simulink model "WEankle_controllerMaarten_2018"  (R2018b)
settings: Solver=FixedStepDiscrete  StartTime=0.0  StopTime=inf  FixedStep=sampleTime  RelTol=1e-3
PreLoadFcn:
  | init
undefined symbols (not defined in the file or in its folder): DiscIntNeverNeededParam, forceplate, Joint_params, sampleTime
libraries: simulink x21, WE2_library x9, dspsigops x6, dspfdesign x3
(part 1 of 4)
settings Model: TCT_ExtModeMexArgs=[130 89 233 2 1 1],16842768  SimulationMode=external  Creator=symbitron  LastModifiedBy=u0088756
settings DataIOCC: LimitDataPoints=on  SaveFormat=StructureWithTime
settings OptimizationCC: LocalBlockOutputs=off
settings DebuggingCC: AllowSymbolicDim=off  SFUnexpectedBacktrackingDiag=warning  SFNoUnconditionalDefaultTransitionDiag=warning  SFExecutionAtInitializationDiag=none
settings HardwareCC: ProdBitPerSizeT=32  ProdBitPerPtrDiffT=32  ProdWordSize=32  ProdHWDeviceType=Specified
settings ModelReferenceCC: PropagateSignalLabelsOutOfModel=off
settings SFSimCC: SimUseLocalCustomCode=off
settings RTWCC: Description=TwinCAT Target  SystemTargetFile=TwinCAT.tlc  GenCodeOnly=on  MakeCommand=make_tct  TemplateMakefile=tct_msbuild.tmf  GenerateReport=on  RTWUseLocalCustomCode=off  TargetLang=C++
settings CodeAppCC: StateflowObjectComments=on
settings STFCustomTargetCC: CompOptLevelCompliant=on  MATLABClassNameForMDSCustomization=Simulink.SoftwareTarget.TargetSpecificTriggerConfigurationBase  GRTInterface=on  SystemTargetFile=TwinCAT.tlc
settings ConfigComp: CovMetricSettings=dw  CovSaveCumulativeToWorkspaceVar=on  CovSaveSingleToWorkspaceVar=on  CovExternalEMLEnable=off

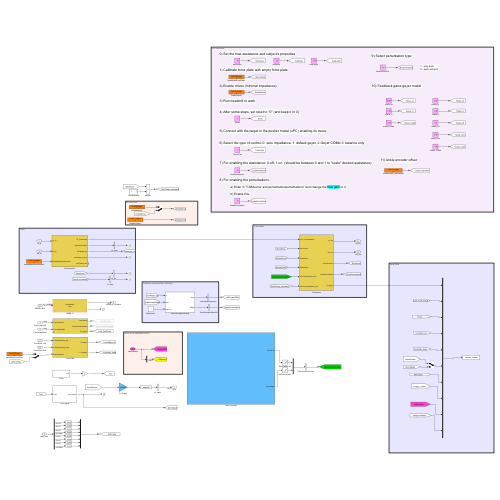
[thumbnail: Simulink's stored preview of the top-level diagram]
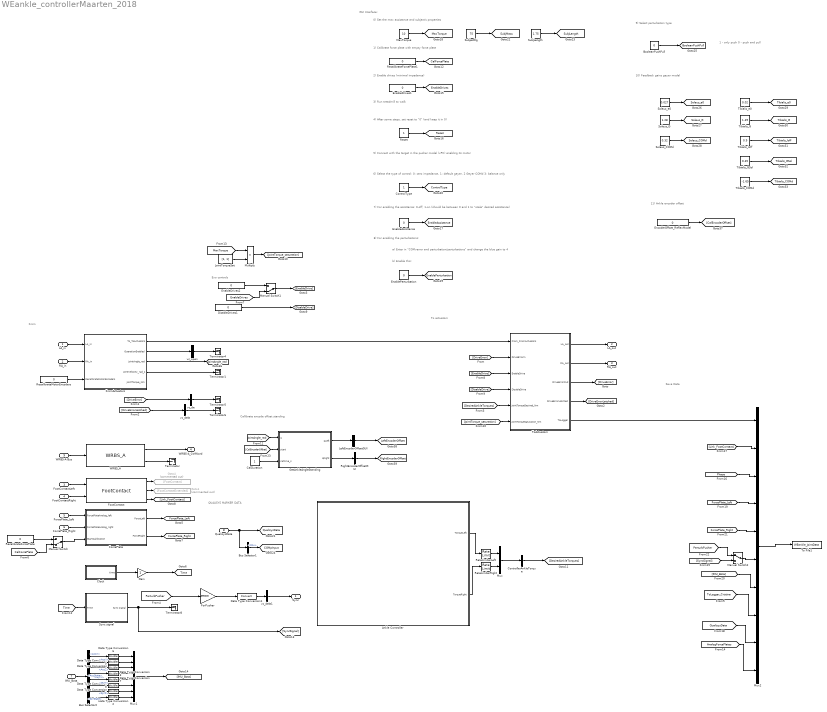
== system WEankle_controllerMaarten_2018 ==
  note: Callibrate encode offset standing
  note: QUALISYS MARKER DATA
  note: GUI Interface:
  note: a) Enter in "COMverror and perturbation/perturbations" and change the blue gain to 4
  note: 1) Calibrate force plate with empty force plate
  note: To actuators
  note: From
  note: Save Data
  note: Exo controls
  note: 2) Enable drives (minimal impedance)
  note: 3) Run treadmill to walk
  note: 4) After some steps, set reset to "0" (and keep it in 0)
  note: 7) For enabling the assistance: 0-off; 1-on (should be between 0 and 1 to "scale" desired assistance)
  note: 0) Set the max assistance and subject's properties
  note: 8) For enabling the perturbations:
  note: b) Enable this:
  note: 5) Connect with the target in the pusher model (xPC) enabling its motor
  note: 6) Select the type of control: 0: zero impedance, 1: default geyer, 2 Geyer COMd 3: balance only
  note: 9) Select perturbation type
  note: 1 - only push
      | 0 - push and pull
  note: 10) Feedback gains geyer model
  note: 11) Ankle encoder offset
  LA_in : Inport  OutDataTypeStr=Bus: WE_InputBus
  RA_in : Inport  Port=2  OutDataTypeStr=Bus: WE_InputBus
  FootContactLeft : Inport  Port=3  OutDataTypeStr=uint32  PortDimensions=1
  FootContactRight : Inport  Port=4  OutDataTypeStr=uint32  PortDimensions=1
  ForcePlate_Left : Inport  Port=5  OutDataTypeStr=Bus: WE_ForcePlateBus
  ForcePlate_Right : Inport  Port=6  OutDataTypeStr=Bus: WE_ForcePlateBus
  IMU_Bota : Inport  Port=7  OutDataTypeStr=Bus: WE_IMUBus
  QualisysData : Inport  Port=8  OutDataTypeStr=Bus: QualisysDataBus
  WRBS-A Bus : Inport  Port=9  OutDataTypeStr=Bus: WE_WRBSABus  BusOutputAsStruct=on
  Ankle Controller : Subsystem
  BooleanPushPull : Constant  Value=0
  Bus Selector1 : BusSelector  OutputSignals=M1x
  Bus Selector2 : BusSelector  OutputSignals=AccX,AccY,AccZ,AccState,GyrX,GyrY,GyrZ,GyrState
  CalDuration : Constant
  Clock : Subsystem
  ControlType : Constant
  ControllerAnkleTorque : Concatenate  NumInputs=1
  Data Type Conversion1 : DataTypeConversion
  Data Type Conversion{2..9} (8 alike) : DataTypeConversion  OutDataTypeStr=double
  DisableDrives1 : Constant  Value=0
      settings: OpenFcn=set_param(gcb,'Value','1');tname = ['toggletimer_' gcb];delete(timerfind('name',tname));t = timer('timerfcn', ['set_param(''',gcb,''',''Value'',''0'')'],'executionmode','singleshot','startdelay',1,'name',tname);start(t);
      mask Display: fprintf('PushToTrigger\n%s',get_param(gcb,'value'))
  EnableAssistance : Constant  Value=0
  EnableDrives1 : Constant  Value=0
      settings: OpenFcn=set_param(gcb,'Value','1');tname = ['toggletimer_' gcb];delete(timerfind('name',tname));t = timer('timerfcn', ['set_param(''',gcb,''',''Value'',''0'')'],'executionmode','singleshot','startdelay',1,'name',tname);start(t);
      mask Display: fprintf('PushToTrigger\n%s',get_param(gcb,'value'))
  EnableDrives2 : Constant  Value=0
      settings: OpenFcn=set_param(gcb,'Value','1');tname = ['toggletimer_' gcb];delete(timerfind('name',tname));t = timer('timerfcn', ['set_param(''',gcb,''',''Value'',''0'')'],'executionmode','singleshot','startdelay',1,'name',tname);start(t);
      mask Display: fprintf('PushToTrigger\n%s',get_param(gcb,'value'))
  EnablePerturbation : Constant  Value=0
  EncoderOffset_ReflexModel : Constant  Value=0
      settings: OpenFcn=set_param(gcb,'Value','1');tname = ['toggletimer_' gcb];delete(timerfind('name',tname));t = timer('timerfcn', ['set_param(''',gcb,''',''Value'',''0'')'],'executionmode','singleshot','startdelay',1,'name',tname);start(t);
      mask Display: fprintf('PushToTrigger\n%s',get_param(gcb,'value'))
  FootContact : WE2_library/FootContact  SystemSampleTime=-1  Latency=0  AutoFrameSizeCalculation=off
  ForPusher : Gain  Gain=695000
  ForcePlate : Subsystem
  FromActuators : Subsystem
  Gain : Gain
  GetAnkleAngleStanding : Subsystem
  Goto1 : Goto  Commented=on  GotoTag=FootContactExtended
  Goto4 : Goto  Commented=on  GotoTag=FootContact
  JointTorqueSat : Constant  Value=[1, 1]
  LeftEncoderOffsetGUI : Concatenate  NumInputs=1
  Manual Switch : ManualSwitch  CurrentSetting=0
  Manual Switch1 : ManualSwitch  CurrentSetting=0
  Manual Switch2 : ManualSwitch
  MaxTorque : Constant  Value=10
  Multiply : Product
  Mux : Mux  Inputs=2
  Mux1 : Mux  Inputs=8
  Mux2 : Mux  Inputs=10
  RateLimiterLeft : RateLimiter  RisingSlewLimit=250  FallingSlewLimit=-250  SampleTimeMode=inherited
  RateLimiterRight : RateLimiter  RisingSlewLimit=250  FallingSlewLimit=-250  SampleTimeMode=inherited
  RecalibrateForcePlate : Constant  Value=0
      settings: OpenFcn=set_param(gcb,'Value','1');tname = ['toggletimer_' gcb];delete(timerfind('name',tname));t = timer('timerfcn', ['set_param(''',gcb,''',''Value'',''0'')'],'executionmode','singleshot','startdelay',1,'name',tname);start(t);
      mask Display: fprintf('PushToTrigger\n%s',get_param(gcb,'value'))
  RecalibrateForcePlate1 : Constant  Value=0
      settings: OpenFcn=set_param(gcb,'Value','1');tname = ['toggletimer_' gcb];delete(timerfind('name',tname));t = timer('timerfcn', ['set_param(''',gcb,''',''Value'',''0'')'],'executionmode','singleshot','startdelay',1,'name',tname);start(t);
      mask Display: fprintf('PushToTrigger\n%s',get_param(gcb,'value'))
  RecalibrateMotorEncoders : Constant  Value=0
      settings: OpenFcn=set_param(gcb,'Value','1');tname = ['toggletimer_' gcb];delete(timerfind('name',tname));t = timer('timerfcn', ['set_param(''',gcb,''',''Value'',''0'')'],'executionmode','singleshot','startdelay',1,'name',tname);start(t);
      mask Display: fprintf('PushToTrigger\n%s',get_param(gcb,'value'))
  Reset : Constant
  RightEncoderOffsetGUI : Concatenate  NumInputs=1
  Soleus_COMd : Constant  Value=0.32
  Soleus_G : Constant  Value=1.28
  Soleus_e0 : Constant  Value=0.027
  SubjLength : Constant  Value=1.75
  SubjectKg : Constant  Value=75
  Sync signal : Subsystem
  Terminator{,1,4..6,8} (6 alike) : Terminator
  Tibialis_COMd : Constant  Value=-1.65
  Tibialis_G : Constant  Value=1.49
  Tibialis_GSol : Constant  Value=0.45
  Tibialis_e0 : Constant  Value=0.02
  Tibialis_loff : Constant  Value=0.9
  To File1 : ToFile  Filename=WEankle_JointData  MatrixName=weankle_jointdata
  ToActuators : Subsystem
  WRBS_A : WE2_library/WRBS_A  SystemSampleTime=-1
  vc_de : Concatenate  NumInputs=1
  vc_dela : Concatenate  NumInputs=1
  vc_dela1 : Concatenate  NumInputs=1
  vc_open : Concatenate  NumInputs=1
  Sync : Outport  OutDataTypeStr=uint16  VectorParamsAs1DForOutWhenUnconnected=off
  LA_out : Outport  Port=2  OutDataTypeStr=Bus: WE_OutputBus  VectorParamsAs1DForOutWhenUnconnected=off
  RA_out : Outport  Port=3  OutDataTypeStr=Bus: WE_OutputBus  VectorParamsAs1DForOutWhenUnconnected=off
  WRBS-A_CtrlWord : Outport  Port=4  OutDataTypeStr=uint16  PortDimensions=1  VectorParamsAs1DForOutWhenUnconnected=off
  tag scope: BooleanPushPull=global, COMpInput=global, CalForcePlate=global, ControlType=global, EnableAssistance=global, EnableDrives=global, EnablePerturbation=global, ForcePlate_Left=global, ForcePlate_Right=global, JointAngle_rad=global, LeftEncoderOffset=global, MaxTorque=global, QualisysData=global, Reset=global, RightEncoderOffset=global, Soleus_COMd=global, Soleus_G=global, Soleus_e0=global, SubjLength=global, SubjMass=global, Tibialis_COMd=global, Tibialis_G=global, Tibialis_GSol=global, Tibialis_e0=global, Tibialis_loff=global, Time=global
  wires:
  ToActuators/1(LA_out) -> LA_out/1
  FromActuators/3(JointAngle_rad) -> [JointAngle_rad]
  FromActuators/4(JointVelocity_rad_s) -> Terminator1/1
  ToActuators/4(DriveErrorLatched) -> [DriveErrorLatched]
  FootContactLeft/1 -> FootContact/1
  FootContactRight/1 -> FootContact/2
  FootContact/1 -> Goto4/1
  FootContact/3 -> [Link_FootContact]
  FootContact/2 -> Goto1/1
  RA_in/1 -> FromActuators/2(RA_in)
  LA_in/1 -> FromActuators/1(LA_in)
  [DriveError] -> ToActuators/2(DriveErrorIn)
  ToActuators/2(RA_out) -> RA_out/1
  FromActuators/1(To_ToActuators) -> ToActuators/1(From_FromActuators)
  FromActuators/2(OperationEnabled) -> vc_open/1
  [DisableDrive] -> ToActuators/4(DisableDrive)
  [JointTorque_saturation] -> ToActuators/6(JointTorqueSaturation_Nm)
  [EnableDrive] -> ToActuators/3(EnableDrive)
  [DesiredAnkleTorques] -> ToActuators/5(JointTorqueDesired_Nm)
  ToActuators/3(DriveErrorOut) -> [DriveError]
  [DriveError] -> vc_de/1
  [DriveErrorLatched] -> vc_dela/1
  RecalibrateMotorEncoders/1 -> FromActuators/3(RecalibrateMotorEncoders)
  vc_open/1 -> Terminator4/1
  vc_de/1 -> Terminator5/1
  vc_dela/1 -> Terminator6/1
  ForcePlate_Left/1 -> ForcePlate/1(ForcePlateAnalog_left)
  ForcePlate_Right/1 -> ForcePlate/2(ForcePlateAnalog_right)
  RecalibrateForcePlate/1 -> Manual Switch/1
  DisableDrives1/1 -> [DisableDrive]
  EnableDrives2/1 -> Manual Switch1/1
  JointTorqueSat/1 -> Multiply/2
  Multiply/1 -> [JointTorque_saturation]
  Data Type Conversion1/1 -> vc_dela1/1
  [Time] -> Sync signal/1(Time)
  Data Type Conversion9/1 -> Mux1/7
  Data Type Conversion3/1 -> Mux1/4
  Data Type Conversion5/1 -> Mux1/2
  Bus Selector2/5 -> Data Type Conversion7/1  "<GyrX>"
  Data Type Conversion8/1 -> Mux1/6
  Data Type Conversion7/1 -> Mux1/5
  Data Type Conversion2/1 -> Mux1/8
  Data Type Conversion6/1 -> Mux1/1
  Data Type Conversion4/1 -> Mux1/3
  Bus Selector2/7 -> Data Type Conversion9/1  "<GyrZ>"
  Bus Selector2/4 -> Data Type Conversion3/1  "<AccState>"
  Bus Selector2/3 -> Data Type Conversion4/1  "<AccZ>"
  Mux1/1 -> [IMU_Bota]
  Bus Selector2/8 -> Data Type Conversion2/1  "<GyrState>"
  Bus Selector2/1 -> Data Type Conversion6/1  "<AccX>"
  Bus Selector2/6 -> Data Type Conversion8/1  "<GyrY>"
  Bus Selector2/2 -> Data Type Conversion5/1  "<AccY>"
  IMU_Bota/1 -> Bus Selector2/1
  Manual Switch2/1 -> Mux2/6
  [IMU_Bota] -> Mux2/7
  ToActuators/5(ToLogger) -> Mux2/1
  [ForcePlate_Left] -> Mux2/4
  [ForcePlate_Right] -> Mux2/5
  Mux2/1 -> To File1/1
  Mux/1 -> ControllerAnkleTorque/1
  ForcePlate/1(ForceLeft) -> [ForcePlate_Left]
  ForcePlate/2(ForceRight) -> [ForcePlate_Right]
  [ToLogger_Cristina] -> Mux2/8
  Clock/1(time) -> Gain/1
  [PerturbPusher] -> ForPusher/1
  vc_dela1/1 -> Sync/1
  ForPusher/1 -> Data Type Conversion1/1
  RateLimiterLeft/1 -> Mux/1
  RateLimiterRight/1 -> Mux/2
  Manual Switch/1 -> ForcePlate/3(StartCalibration)
  [CalForcePlate] -> Manual Switch/2
  RecalibrateForcePlate1/1 -> [CalForcePlate]
  Manual Switch1/1 -> [EnableDrive]
  [EnableDrives] -> Manual Switch1/2
  EnableDrives1/1 -> [EnableDrives]
  Reset/1 -> [Reset]
  EnableAssistance/1 -> [EnableAssistance]
  MaxTorque/1 -> [MaxTorque]
  [MaxTorque] -> Multiply/1
  EnablePerturbation/1 -> [EnablePerturbation]
  ControlType/1 -> [ControlType]
  SubjectKg/1 -> [SubjMass]
  SubjLength/1 -> [SubjLength]
  Bus Selector1/1 -> [COMpInput]  "<M1x>"
  QualisysData/1 -> Bus Selector1/1, [QualisysData]
  [QualisysData] -> Mux2/9
  [AnalogForcePlates] -> Mux2/10
  [PerturbPusher] -> Manual Switch2/1
  [SyncSignal] -> Manual Switch2/2
  Sync signal/1(Sync signal) -> [SyncSignal], Terminator8/1
  BooleanPushPull/1 -> [BooleanPushPull]
  Soleus_e0/1 -> [Soleus_e0]
  Soleus_G/1 -> [Soleus_G]
  Soleus_COMd/1 -> [Soleus_COMd]
  Tibialis_e0/1 -> [Tibialis_e0]
  Tibialis_G/1 -> [Tibialis_G]
  Tibialis_loff/1 -> [Tibialis_loff]
  Tibialis_GSol/1 -> [Tibialis_GSol]
  Tibialis_COMd/1 -> [Tibialis_COMd]
  Gain/1 -> [Time]
  [Link_FootContact] -> Mux2/2
  [Phase] -> Mux2/3
  ControllerAnkleTorque/1 -> [DesiredAnkleTorques]
  WRBS_A/2 -> Terminator/1
  WRBS-A Bus/1 -> WRBS_A/1
  WRBS_A/1 -> WRBS-A_CtrlWord/1
  Ankle Controller/1(TorqueLeft) -> RateLimiterLeft/1
  Ankle Controller/2(TorqueRight) -> RateLimiterRight/1
  EncoderOffset_ReflexModel/1 -> [CalEncoderOffset]
  [JointAngle_rad] -> GetAnkleAngleStanding/1(q)
  [CalEncoderOffset] -> GetAnkleAngleStanding/2(start)
  CalDuration/1 -> GetAnkleAngleStanding/3(caltime_s)
  GetAnkleAngleStanding/1(qLeft) -> LeftEncoderOffsetGUI/1
  GetAnkleAngleStanding/2(qRight) -> RightEncoderOffsetGUI/1
  LeftEncoderOffsetGUI/1 -> [LeftEncoderOffset]
  RightEncoderOffsetGUI/1 -> [RightEncoderOffset]

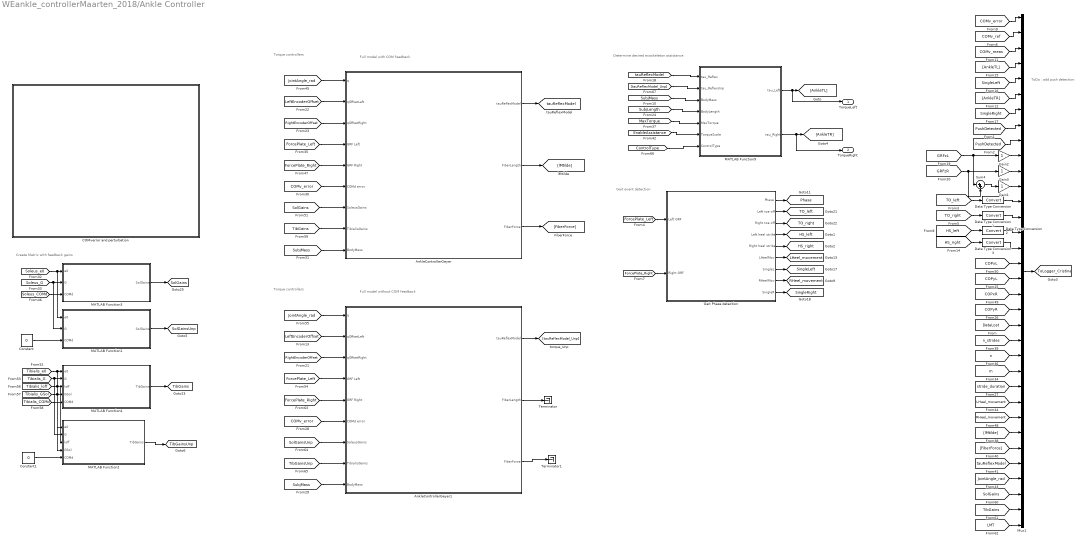
== system WEankle_controllerMaarten_2018/Ankle Controller ==
  note: Gait event detection
  note: Determine desired exoskeleton assistance
  note: Full model with COM feedback
  note: Create Matrix with feedback gains
  note: ToDo : add push detection
  note: Torque controllers
  note: Full model without COM feedback
  note: Torque controllers
  AnkleControllerGeyer : Subsystem
  AnkleControllerGeyer1 : Subsystem
  COMverror and perturbation : Subsystem
  Constant : Constant  Value=0
  Constant1 : Constant  Value=0
  Data Type Conversion{,1..3} (4 alike) : DataTypeConversion
  Gain1 : Gain
  Gain2 : Gain
  Gain3 : Gain
  Gait Phase detection : Subsystem
  MATLAB Function1 : MATLAB Function  TreatAsAtomicUnit=on
  MATLAB Function2 : MATLAB Function  TreatAsAtomicUnit=on
  MATLAB Function3 : MATLAB Function  TreatAsAtomicUnit=on
  MATLAB Function4 : MATLAB Function  TreatAsAtomicUnit=on
  MATLAB Function9 : MATLAB Function  TreatAsAtomicUnit=on
  Mux1 : Mux  Inputs=34
  Sum4 : Sum  Inputs=|++
  Terminator : Terminator
  Terminator1 : Terminator
  TorqueLeft : Outport
  TorqueRight : Outport  Port=2
  tag scope: HS_left=global, HS_right=global, LHeel_movement=global, Phase=global, RHeel_movement=global, SingleLeft=global, SingleRight=global, SolGains=global, SolGainsUnp=global, TO_left=global, TO_right=global, TibGains=global, TibGainsUnp=global, ToLogger_Cristina=global, tauReflexModel=global
  wires:
  [COMv_error] -> Mux1/1
  [COMv_ref] -> Mux1/2
  [COMv_meas] -> Mux1/3
  [AnkleTL] -> Mux1/4
  [AnkleTR] -> Mux1/6
  [SingleRight] -> Mux1/7
  [SingleLeft] -> Mux1/5
  Sum4/1 -> Gain1/1
  [GRFzL] -> Gain2/1, Sum4/1
  [GRFzR] -> Gain3/1, Sum4/2
  [HS_right] -> Data Type Conversion3/1
  [HS_left] -> Data Type Conversion2/1
  [TO_right] -> Data Type Conversion1/1
  [TO_left] -> Data Type Conversion/1
  [RHeel_movement] -> Mux1/27
  [LHeel_movement] -> Mux1/26
  [stride_duration] -> Mux1/25
  [m] -> Mux1/24
  [n] -> Mux1/23
  [n_strides] -> Mux1/22
  [DataLost] -> Mux1/21
  [COPyR] -> Mux1/20
  [COPxR] -> Mux1/19
  [COPyL] -> Mux1/18
  [COPxL] -> Mux1/17
  Data Type Conversion3/1 -> Mux1/16
  Data Type Conversion2/1 -> Mux1/15
  Data Type Conversion1/1 -> Mux1/14
  Data Type Conversion/1 -> Mux1/13
  Gain1/1 -> Mux1/12
  Gain3/1 -> Mux1/11
  Gain2/1 -> Mux1/10
  Mux1/1 -> [ToLogger_Cristina]
  [lMtilde] -> Mux1/28
  [FiberForce] -> Mux1/29
  [tauReflexModel] -> Mux1/30
  [JointAngle_rad] -> Mux1/31
  [SolGains] -> Mux1/32
  [TibGains] -> Mux1/33
  [LMT] -> Mux1/34
  [ForcePlate_Left] -> Gait Phase detection/1(Left GRF)
  [ForcePlate_Right] -> Gait Phase detection/2(Right GRF)
  Gait Phase detection/1(Phase) -> [Phase]
  Gait Phase detection/2(Left toe off) -> [TO_left]
  Gait Phase detection/3(Right toe off) -> [TO_right]
  Gait Phase detection/4(Left heel strike) -> [HS_left]
  Gait Phase detection/5(Right heel strike) -> [HS_right]
  Gait Phase detection/6(LHeelMov) -> [LHeel_movement]
  Gait Phase detection/7(SingleL) -> [SingleLeft]
  Gait Phase detection/8(RHeelMov) -> [RHeel_movement]
  Gait Phase detection/9(SingleR) -> [SingleRight]
  [JointAngle_rad] -> AnkleControllerGeyer/1(q)
  [LeftEncoderOffset] -> AnkleControllerGeyer/2(qOffsetLeft)
  [RightEncoderOffset] -> AnkleControllerGeyer/3(qOffsetRight)
  [ForcePlate_Left] -> AnkleControllerGeyer/4(GRF Left)
  [ForcePlate_Right] -> AnkleControllerGeyer/5(GRF Right)
  [COMv_error] -> AnkleControllerGeyer/6(COMd error)
  [SolGains] -> AnkleControllerGeyer/7(SoleusGains)
  [TibGains] -> AnkleControllerGeyer/8(TibialisGains)
  [SubjMass] -> AnkleControllerGeyer/9(BodyMass)
  [PushDetected] -> Mux1/8
  [PushDetected] -> Mux1/9
  [Tibialis_e0] -> MATLAB Function2/1(e0), MATLAB Function4/1(e0)
  [Soleus_e0] -> MATLAB Function1/1(e0), MATLAB Function3/1(e0)
  [Tibialis_loff] -> MATLAB Function2/3(loff), MATLAB Function4/3(loff)
  MATLAB Function3/1(SolGains) -> [SolGains]
  [Tibialis_COMd] -> MATLAB Function4/5(COMd)
  [Soleus_G] -> MATLAB Function3/2(G), MATLAB Function1/2(G)
  [Tibialis_G] -> MATLAB Function4/2(G), MATLAB Function2/2(G)
  [Tibialis_GSol] -> MATLAB Function2/4(GSol), MATLAB Function4/4(GSol)
  [Soleus_COMd] -> MATLAB Function3/3(COMd)
  MATLAB Function4/1(TibGains) -> [TibGains]
  [tauReflexModel] -> MATLAB Function9/1(tau_Reflex)
  MATLAB Function9/2(tau_Right) -> TorqueRight/1, [AnkleTR]
  [SubjMass] -> MATLAB Function9/3(BodyMass)
  [EnableAssistance] -> MATLAB Function9/6(TorqueScale)
  MATLAB Function9/1(tau_Left) -> TorqueLeft/1, [AnkleTL]
  AnkleControllerGeyer/2(FiberLength) -> [lMtilde]
  AnkleControllerGeyer/3(FiberForce) -> [FiberForce]
  AnkleControllerGeyer/1(tauReflexModel) -> [tauReflexModel]
  [MaxTorque] -> MATLAB Function9/5(MaxTorque)
  [SubjLength] -> MATLAB Function9/4(BodyLength)
  Constant/1 -> MATLAB Function1/3(COMd)
  MATLAB Function1/1(SolGains) -> [SolGainsUnp]
  Constant1/1 -> MATLAB Function2/5(COMd)
  MATLAB Function2/1(TibGains) -> [TibGainsUnp]
  [SubjMass] -> AnkleControllerGeyer1/9(BodyMass)
  [RightEncoderOffset] -> AnkleControllerGeyer1/3(qOffsetRight)
  [SolGainsUnp] -> AnkleControllerGeyer1/7(SoleusGains)
  [ForcePlate_Right] -> AnkleControllerGeyer1/5(GRF Right)
  [COMv_error] -> AnkleControllerGeyer1/6(COMd error)
  [TibGainsUnp] -> AnkleControllerGeyer1/8(TibialisGains)
  [JointAngle_rad] -> AnkleControllerGeyer1/1(q)
  [LeftEncoderOffset] -> AnkleControllerGeyer1/2(qOffsetLeft)
  AnkleControllerGeyer1/1(tauReflexModel) -> [tauReflexModel_Unp]
  AnkleControllerGeyer1/3(FiberForce) -> Terminator1/1
  AnkleControllerGeyer1/2(FiberLength) -> Terminator/1
  [ForcePlate_Left] -> AnkleControllerGeyer1/4(GRF Left)
  [ControlType] -> MATLAB Function9/7(ControlType)
  [tauReflexModel_Unp] -> MATLAB Function9/2(tau_ReflexUnp)

== system WEankle_controllerMaarten_2018/Clock ==
  Constant : Constant
  Discrete-Time Integrator : DiscreteIntegrator  SampleTime=-1  ICPrevOutput=DiscIntNeverNeededParam  ICPrevScaledInput=DiscIntNeverNeededParam
  time : Outport  VectorParamsAs1DForOutWhenUnconnected=off
  wires:
  Discrete-Time Integrator/1 -> time/1
  Constant/1 -> Discrete-Time Integrator/1

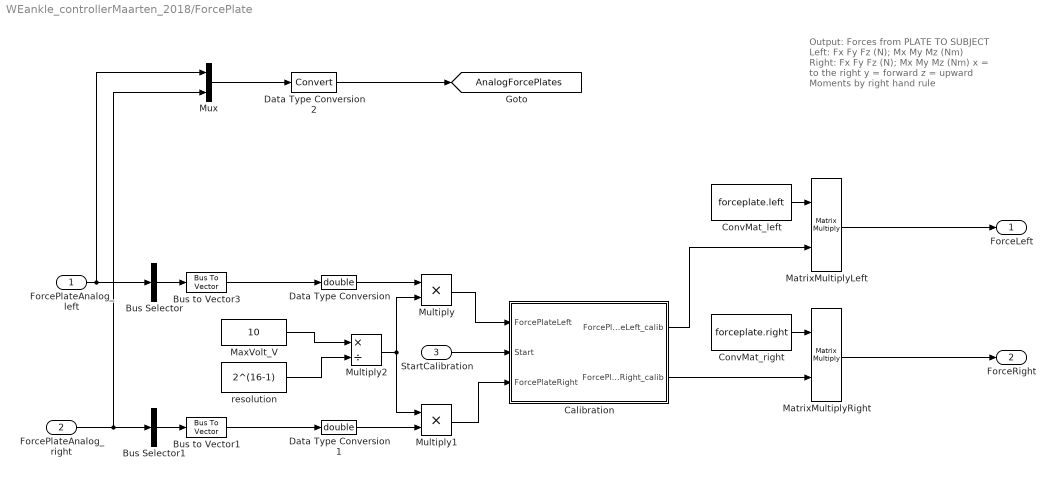
== system WEankle_controllerMaarten_2018/ForcePlate ==
  note: Output:
      | Forces from PLATE TO SUBJECT
      | Left: Fx Fy Fz (N); Mx My Mz (Nm)
      | Right: Fx Fy Fz (N); Mx My Mz (Nm)
      | x = to the right
      | y = forward
      | z = upward
      | Moments by right hand rule
  ForcePlateAnalog_left : Inport
  ForcePlateAnalog_right : Inport  Port=2
  StartCalibration : Inport  Port=3
  Bus Selector : BusSelector  OutputSignals=Input1,Input2,Input3,Input4,Input5,Input6,Input7  OutputAsBus=on
  Bus Selector1 : BusSelector  OutputSignals=Input1,Input2,Input3,Input4,Input5,Input6,Input7  OutputAsBus=on
  Bus to Vector1 : BusToVector
  Bus to Vector3 : BusToVector
  Calibration : Subsystem
  ConvMat_left : Constant  Value=forceplate.left  VectorParams1D=off
  ConvMat_right : Constant  Value=forceplate.right  VectorParams1D=off
  Data Type Conversion : DataTypeConversion  OutDataTypeStr=double
  Data Type Conversion1 : DataTypeConversion  OutDataTypeStr=double
  Data Type Conversion2 : DataTypeConversion
  MatrixMultiplyLeft : Product  Multiplication=Matrix(*)
  MatrixMultiplyRight : Product  Multiplication=Matrix(*)
  MaxVolt_V : Constant  Value=10
  Multiply : Product
  Multiply1 : Product
  Multiply2 : Product  Inputs=*/
  Mux : Mux  Inputs=2
  resolution : Constant  Value=2^(16-1)
  ForceLeft : Outport  VectorParamsAs1DForOutWhenUnconnected=off
  ForceRight : Outport  Port=2  VectorParamsAs1DForOutWhenUnconnected=off
  tag scope: AnalogForcePlates=global
  wires:
  ForcePlateAnalog_left/1 -> Mux/1, Bus Selector/1
  ForcePlateAnalog_right/1 -> Mux/2, Bus Selector1/1
  Data Type Conversion/1 -> Multiply/1
  Data Type Conversion1/1 -> Multiply1/2
  Multiply2/1 -> Multiply1/1, Multiply/2
  Multiply/1 -> Calibration/1(ForcePlateLeft)
  Multiply1/1 -> Calibration/3(ForcePlateRight)
  ConvMat_left/1 -> MatrixMultiplyLeft/1
  MatrixMultiplyLeft/1 -> ForceLeft/1
  MatrixMultiplyRight/1 -> ForceRight/1
  ConvMat_right/1 -> MatrixMultiplyRight/1
  Bus to Vector3/1 -> Data Type Conversion/1
  Bus to Vector1/1 -> Data Type Conversion1/1
  Bus Selector/1 -> Bus to Vector3/1
  Bus Selector1/1 -> Bus to Vector1/1
  resolution/1 -> Multiply2/2
  MaxVolt_V/1 -> Multiply2/1
  StartCalibration/1 -> Calibration/2(Start)
  Calibration/1(ForcePlateLeft_calib) -> MatrixMultiplyLeft/2
  Calibration/2(ForcePlateRight_calib) -> MatrixMultiplyRight/2
  Mux/1 -> Data Type Conversion2/1
  Data Type Conversion2/1 -> [AnalogForcePlates]

== system WEankle_controllerMaarten_2018/FromActuators ==
  LA_in : Inport  OutDataTypeStr=Bus: WE_InputBus
  RA_in : Inport  Port=2  OutDataTypeStr=Bus: WE_InputBus
  RecalibrateMotorEncoders : Inport  Port=3
  LA : WE2_library/FromActuator  ActuatorStruct=Joint_params.LA
  Logical Operator2 : Logic  Operator=OR  Inputs=1  AllPortsSameDT=off  OutDataTypeStr=boolean
  Mux{11..14} (4 alike) : Mux  Inputs=2
  RA : Subsystem  AncestorBlock=WE2_library/FromActuator  mask{ActuatorStruct=Joint_params.RA}
      mask prompts: ActuatorStruct "Acutator Struct"
  Vector Concatenate2 : Concatenate
  To_ToActuators : Outport  VectorParamsAs1DForOutWhenUnconnected=off
  OperationEnabled : Outport  Port=2  VectorParamsAs1DForOutWhenUnconnected=off
  JointAngle_rad : Outport  Port=3  VectorParamsAs1DForOutWhenUnconnected=off
  JointVelocity_rad_s : Outport  Port=4  VectorParamsAs1DForOutWhenUnconnected=off
  JointTorque_Nm : Outport  Port=5  VectorParamsAs1DForOutWhenUnconnected=off
  wires:
  RecalibrateMotorEncoders/1 -> Logical Operator2/1
  Mux14/1 -> JointTorque_Nm/1
  Mux13/1 -> JointVelocity_rad_s/1
  Mux12/1 -> JointAngle_rad/1
  Mux11/1 -> OperationEnabled/1
  Vector Concatenate2/1 -> To_ToActuators/1
  RA/5(JointTorque_Nm) -> Mux14/2
  LA/5 -> Mux14/1
  RA/4(JointVelocity_rad_s) -> Mux13/2
  LA/4 -> Mux13/1
  RA/3(JointAngle_rad) -> Mux12/2
  LA/3 -> Mux12/1
  RA/2(OperationEnabled) -> Mux11/2
  LA/2 -> Mux11/1
  RA/1(To_ToActuator) -> Vector Concatenate2/2
  LA/1 -> Vector Concatenate2/1
  Logical Operator2/1 -> RA/2(RecalibrateMotorEncoder), LA/2
  LA_in/1 -> LA/1
  RA_in/1 -> RA/1(TwinCATSignalsIn)

== system WEankle_controllerMaarten_2018/GetAnkleAngleStanding ==
  q : Inport
  start : Inport  Port=2
  caltime_s : Inport  Port=3
  MATLAB Function : MATLAB Function  TreatAsAtomicUnit=on
  MATLAB Function1 : MATLAB Function  TreatAsAtomicUnit=on
  Selector1 : Selector  InputPortWidth=6  IndexOptions=Index vector (dialog)  Indices=2  OutputSizes=1
  Selector4 : Selector  InputPortWidth=6  IndexOptions=Index vector (dialog)  Indices=1  OutputSizes=1
  qLeft : Outport
  qRight : Outport  Port=2
  wires:
  MATLAB Function1/1(qOff) -> qRight/1
  Selector4/1 -> MATLAB Function/1(q)
  caltime_s/1 -> MATLAB Function/3(caltime_s), MATLAB Function1/3(caltime_s)
  Selector1/1 -> MATLAB Function1/1(q)
  q/1 -> Selector4/1, Selector1/1
  MATLAB Function/1(qOff) -> qLeft/1
  start/1 -> MATLAB Function/2(start), MATLAB Function1/2(start)

== system WEankle_controllerMaarten_2018/Sync signal ==
  Time : Inport
  Compare To Zero : simulink/Logic and Bit Operations/Compare To Zero  relop=>=  OutDataTypeStr=boolean
  Constant2 : Constant  Value=0.1
  Gain : Gain  Gain=1000
  Sample and Hold : dspsigops/Sample and Hold  trig=Rising edge  initCond=0  latchinput=off
  Sample and Hold1 : dspsigops/Sample and Hold  trig=Rising edge  initCond=0  latchinput=off
  Sum : Sum  Inputs=--+
  Uniform Random Number : UniformRandomNumber  SampleTime=0.001
  Unit Delay : UnitDelay  SampleTime=-1  HasFrameUpgradeWarning=on
  Sync signal : Outport  VectorParamsAs1DForOutWhenUnconnected=off
  wires:
  Time/1 -> Sum/3, Sample and Hold/1
  Sample and Hold/1 -> Sum/2
  Unit Delay/1 -> Sample and Hold1/Trigger, Sample and Hold/Trigger
  Constant2/1 -> Sum/1
  Sum/1 -> Compare To Zero/1
  Compare To Zero/1 -> Unit Delay/1
  Uniform Random Number/1 -> Sample and Hold1/1
  Sample and Hold1/1 -> Gain/1
  Gain/1 -> Sync signal/1

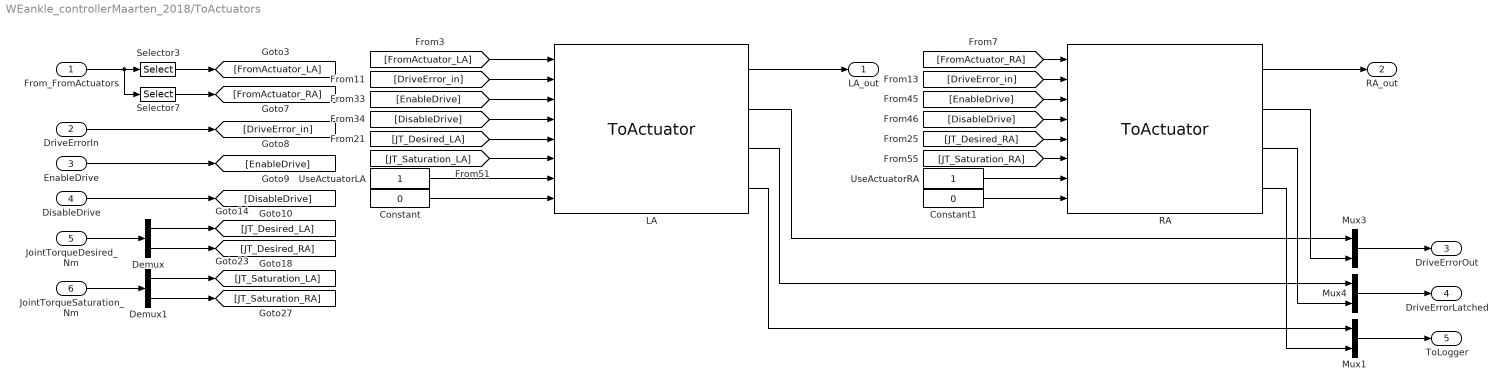
== system WEankle_controllerMaarten_2018/ToActuators ==
  From_FromActuators : Inport  OutDataTypeStr=Bus: WE_ToToActuatorBus
  DriveErrorIn : Inport  Port=2
  EnableDrive : Inport  Port=3
  DisableDrive : Inport  Port=4
  JointTorqueDesired_Nm : Inport  Port=5
  JointTorqueSaturation_Nm : Inport  Port=6
  Constant : Constant  Value=0
  Constant1 : Constant  Value=0
  Demux : Demux  Outputs=2
  Demux1 : Demux  Outputs=2
  LA : WE2_library/ToActuator  side=Left  ActuatorStruct=Joint_params.LA
  Mux1 : Mux  Inputs=2
  Mux3 : Mux  Inputs=2
  Mux4 : Mux  Inputs=2
  RA : WE2_library/ToActuator  side=Right  ActuatorStruct=Joint_params.RA
  Selector3 : Selector  InputPortWidth=2  IndexOptions=Index vector (dialog)  Indices=1  OutputSizes=1
  Selector7 : Selector  InputPortWidth=2  IndexOptions=Index vector (dialog)  Indices=2  OutputSizes=1
  UseActuatorLA : Constant  OutDataTypeStr=double
      settings: OpenFcn=|
      | b = get_param(gcb,'value');
      | if (strcmp(b,'1')),
      |   set_param (gcb,'value','0');
      | else
      |   set_param(gcb,'value','1');
      | end;
  UseActuatorRA : Constant  OutDataTypeStr=double
      settings: OpenFcn=|
      | b = get_param(gcb,'value');
      | if (strcmp(b,'1')),
      |   set_param (gcb,'value','0');
      | else
      |   set_param(gcb,'value','1');
      | end;
  LA_out : Outport  VectorParamsAs1DForOutWhenUnconnected=off
  RA_out : Outport  Port=2  VectorParamsAs1DForOutWhenUnconnected=off
  DriveErrorOut : Outport  Port=3  VectorParamsAs1DForOutWhenUnconnected=off
  DriveErrorLatched : Outport  Port=4  VectorParamsAs1DForOutWhenUnconnected=off
  ToLogger : Outport  Port=5  VectorParamsAs1DForOutWhenUnconnected=off
  wires:
  UseActuatorRA/1 -> RA/7
  UseActuatorLA/1 -> LA/7
  Mux1/1 -> ToLogger/1
  Mux4/1 -> DriveErrorLatched/1
  Mux3/1 -> DriveErrorOut/1
  RA/4 -> Mux1/2
  LA/4 -> Mux1/1
  LA/3 -> Mux4/1
  LA/2 -> Mux3/1
  RA/3 -> Mux4/2
  RA/2 -> Mux3/2
  DisableDrive/1 -> [DisableDrive]
  [JT_Saturation_RA] -> RA/6
  [DisableDrive] -> RA/4
  [EnableDrive] -> RA/3
  [JT_Desired_RA] -> RA/5
  [JT_Saturation_LA] -> LA/6
  [JT_Desired_LA] -> LA/5
  Demux1/2 -> [JT_Saturation_RA]
  JointTorqueSaturation_Nm/1 -> Demux1/1
  Demux1/1 -> [JT_Saturation_LA]
  [DisableDrive] -> LA/4
  [EnableDrive] -> LA/3
  Demux/2 -> [JT_Desired_RA]
  JointTorqueDesired_Nm/1 -> Demux/1
  Demux/1 -> [JT_Desired_LA]
  EnableDrive/1 -> [EnableDrive]
  [DriveError_in] -> LA/2
  [DriveError_in] -> RA/2
  DriveErrorIn/1 -> [DriveError_in]
  From_FromActuators/1 -> Selector7/1, Selector3/1
  [FromActuator_LA] -> LA/1
  [FromActuator_RA] -> RA/1
  Selector7/1 -> [FromActuator_RA]
  Selector3/1 -> [FromActuator_LA]
  Constant/1 -> LA/8
  Constant1/1 -> RA/8
  LA/1 -> LA_out/1
  RA/1 -> RA_out/1

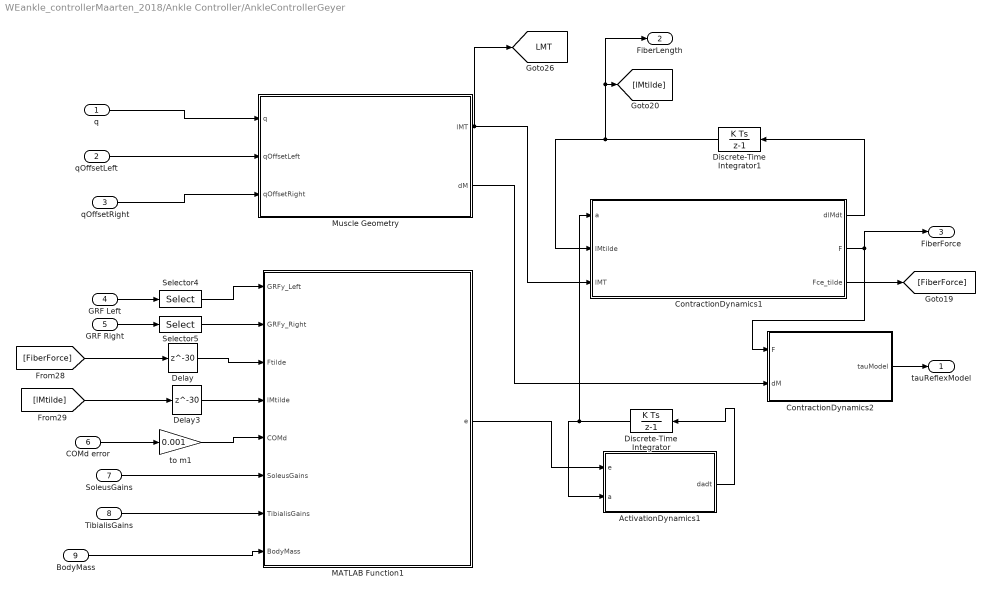
== system WEankle_controllerMaarten_2018/Ankle Controller/AnkleControllerGeyer ==
  q : Inport
  qOffsetLeft : Inport  Port=2
  qOffsetRight : Inport  Port=3
  GRF Left : Inport  Port=4
  GRF Right : Inport  Port=5
  COMd error : Inport  Port=6
  SoleusGains : Inport  Port=7
  TibialisGains : Inport  Port=8
  BodyMass : Inport  Port=9
  ActivationDynamics1 : MATLAB Function  TreatAsAtomicUnit=on
  ContractionDynamics1 : MATLAB Function  TreatAsAtomicUnit=on
  ContractionDynamics2 : MATLAB Function  TreatAsAtomicUnit=on
  Delay : Delay  DelayLength=30  InitialCondition=0
  Delay3 : Delay  DelayLength=30  InitialCondition=1
  Discrete-Time Integrator : DiscreteIntegrator  InitialCondition=[0.2; 0.2; 0.2; 0.2]  SampleTime=-1  ICPrevOutput=DiscIntNeverNeededParam  ICPrevScaledInput=DiscIntNeverNeededParam
  Discrete-Time Integrator1 : DiscreteIntegrator  InitialCondition=[0.7; 1; 0.7; 1]  SampleTime=-1  LimitOutput=on  UpperSaturationLimit=[1.3; 1.3; 1.3; 1.3]  LowerSaturationLimit=[0.5; 0.5; 0.5; 0.5]  ICPrevOutput=DiscIntNeverNeededParam  ICPrevScaledInput=DiscIntNeverNeededParam
  MATLAB Function1 : MATLAB Function  TreatAsAtomicUnit=on
  Muscle Geometry : MATLAB Function  TreatAsAtomicUnit=on
  Selector4 : Selector  InputPortWidth=6  IndexOptions=Index vector (dialog)  Indices=3  OutputSizes=1
  Selector5 : Selector  InputPortWidth=6  IndexOptions=Index vector (dialog)  Indices=3  OutputSizes=1
  to m1 : Gain  Gain=0.001
  tauReflexModel : Outport  VectorParamsAs1DForOutWhenUnconnected=off
  FiberLength : Outport  Port=2  VectorParamsAs1DForOutWhenUnconnected=off
  FiberForce : Outport  Port=3  VectorParamsAs1DForOutWhenUnconnected=off
  tag scope: LMT=global
  wires:
  GRF Left/1 -> Selector4/1
  Muscle Geometry/1(lMT) -> [LMT], ContractionDynamics1/3(lMT)
  ActivationDynamics1/1(dadt) -> Discrete-Time Integrator/1
  Muscle Geometry/2(dM) -> ContractionDynamics2/2(dM)
  Discrete-Time Integrator/1 -> ContractionDynamics1/1(a), ActivationDynamics1/2(a)
  Discrete-Time Integrator1/1 -> FiberLength/1, [lMtilde], ContractionDynamics1/2(lMtilde)
  Selector4/1 -> MATLAB Function1/1(GRFy_Left)
  TibialisGains/1 -> MATLAB Function1/7(TibialisGains)
  Delay/1 -> MATLAB Function1/3(Ftilde)
  ContractionDynamics1/3(Fce_tilde) -> [FiberForce]
  Delay3/1 -> MATLAB Function1/4(lMtilde)
  Selector5/1 -> MATLAB Function1/2(GRFy_Right)
  [lMtilde] -> Delay3/1
  BodyMass/1 -> MATLAB Function1/8(BodyMass)
  [FiberForce] -> Delay/1
  ContractionDynamics2/1(tauModel) -> tauReflexModel/1
  ContractionDynamics1/1(dlMdt) -> Discrete-Time Integrator1/1
  to m1/1 -> MATLAB Function1/5(COMd)
  ContractionDynamics1/2(F) -> FiberForce/1, ContractionDynamics2/1(F)
  MATLAB Function1/1(e) -> ActivationDynamics1/1(e)
  SoleusGains/1 -> MATLAB Function1/6(SoleusGains)
  qOffsetLeft/1 -> Muscle Geometry/2(qOffsetLeft)
  COMd error/1 -> to m1/1
  q/1 -> Muscle Geometry/1(q)
  qOffsetRight/1 -> Muscle Geometry/3(qOffsetRight)
  GRF Right/1 -> Selector5/1

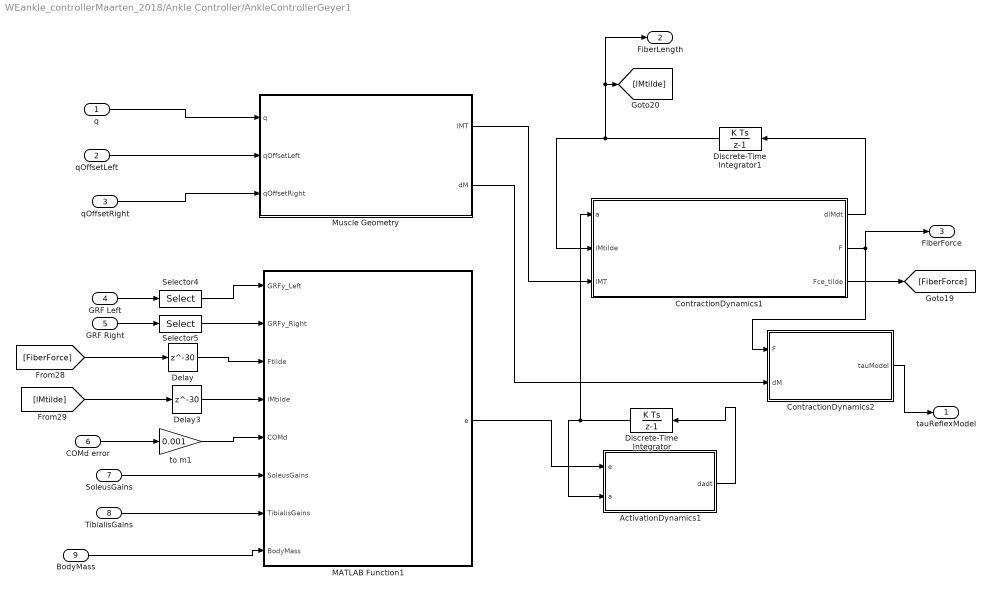
== system WEankle_controllerMaarten_2018/Ankle Controller/AnkleControllerGeyer1 ==
  q : Inport
  qOffsetLeft : Inport  Port=2
  qOffsetRight : Inport  Port=3
  GRF Left : Inport  Port=4
  GRF Right : Inport  Port=5
  COMd error : Inport  Port=6
  SoleusGains : Inport  Port=7
  TibialisGains : Inport  Port=8
  BodyMass : Inport  Port=9
  ActivationDynamics1 : MATLAB Function  TreatAsAtomicUnit=on
  ContractionDynamics1 : MATLAB Function  TreatAsAtomicUnit=on
  ContractionDynamics2 : MATLAB Function  TreatAsAtomicUnit=on
  Delay : Delay  DelayLength=30  InitialCondition=0
  Delay3 : Delay  DelayLength=30  InitialCondition=1
  Discrete-Time Integrator : DiscreteIntegrator  InitialCondition=[0.2; 0.2; 0.2; 0.2]  SampleTime=-1  ICPrevOutput=DiscIntNeverNeededParam  ICPrevScaledInput=DiscIntNeverNeededParam
  Discrete-Time Integrator1 : DiscreteIntegrator  InitialCondition=[0.7; 1; 0.7; 1]  SampleTime=-1  LimitOutput=on  UpperSaturationLimit=[1.3; 1.3; 1.3; 1.3]  LowerSaturationLimit=[0.5; 0.5; 0.5; 0.5]  ICPrevOutput=DiscIntNeverNeededParam  ICPrevScaledInput=DiscIntNeverNeededParam
  MATLAB Function1 : MATLAB Function  TreatAsAtomicUnit=on
  Muscle Geometry : MATLAB Function  TreatAsAtomicUnit=on
  Selector4 : Selector  InputPortWidth=6  IndexOptions=Index vector (dialog)  Indices=3  OutputSizes=1
  Selector5 : Selector  InputPortWidth=6  IndexOptions=Index vector (dialog)  Indices=3  OutputSizes=1
  to m1 : Gain  Gain=0.001
  tauReflexModel : Outport  VectorParamsAs1DForOutWhenUnconnected=off
  FiberLength : Outport  Port=2  VectorParamsAs1DForOutWhenUnconnected=off
  FiberForce : Outport  Port=3  VectorParamsAs1DForOutWhenUnconnected=off
  wires:
  GRF Left/1 -> Selector4/1
  Muscle Geometry/1(lMT) -> ContractionDynamics1/3(lMT)
  ActivationDynamics1/1(dadt) -> Discrete-Time Integrator/1
  Muscle Geometry/2(dM) -> ContractionDynamics2/2(dM)
  Discrete-Time Integrator/1 -> ContractionDynamics1/1(a), ActivationDynamics1/2(a)
  Discrete-Time Integrator1/1 -> FiberLength/1, [lMtilde], ContractionDynamics1/2(lMtilde)
  Selector4/1 -> MATLAB Function1/1(GRFy_Left)
  TibialisGains/1 -> MATLAB Function1/7(TibialisGains)
  Delay/1 -> MATLAB Function1/3(Ftilde)
  ContractionDynamics1/3(Fce_tilde) -> [FiberForce]
  Delay3/1 -> MATLAB Function1/4(lMtilde)
  Selector5/1 -> MATLAB Function1/2(GRFy_Right)
  [lMtilde] -> Delay3/1
  BodyMass/1 -> MATLAB Function1/8(BodyMass)
  [FiberForce] -> Delay/1
  ContractionDynamics2/1(tauModel) -> tauReflexModel/1
  ContractionDynamics1/1(dlMdt) -> Discrete-Time Integrator1/1
  to m1/1 -> MATLAB Function1/5(COMd)
  ContractionDynamics1/2(F) -> FiberForce/1, ContractionDynamics2/1(F)
  MATLAB Function1/1(e) -> ActivationDynamics1/1(e)
  SoleusGains/1 -> MATLAB Function1/6(SoleusGains)
  qOffsetLeft/1 -> Muscle Geometry/2(qOffsetLeft)
  COMd error/1 -> to m1/1
  q/1 -> Muscle Geometry/1(q)
  qOffsetRight/1 -> Muscle Geometry/3(qOffsetRight)
  GRF Right/1 -> Selector5/1

== system WEankle_controllerMaarten_2018/Ankle Controller/COMverror and perturbation ==
  COMvError : Subsystem
  Data Type Conversion : DataTypeConversion
  TriggerPerturbation : Subsystem
  tag scope: COMv_error=global, COMv_meas=global, COMv_ref=global, PerturbPusher=global, PushDetected=global
  wires:
  [TO_left] -> Data Type Conversion/1
  Data Type Conversion/1 -> COMvError/2(trigger)
  [Time] -> COMvError/1(Signaltime)
  [COMpInput] -> COMvError/3(xPosCOM)
  COMvError/4(COMv_error) -> [COMv_error]  "COMvError"
  COMvError/2(COMv_meas) -> [COMv_meas]  "COMvMeas"
  [EnablePerturbation] -> TriggerPerturbation/1(In1)
  [BooleanPushPull] -> TriggerPerturbation/2(In2)
  [SingleRight] -> TriggerPerturbation/3(SingleR)
  [SingleLeft] -> TriggerPerturbation/4(SingleL)
  [Phase] -> TriggerPerturbation/5(In5)
  [ForcePlate_Left] -> TriggerPerturbation/6(In6)
  TriggerPerturbation/1(PerturbationTrigger) -> [PerturbPusher]
  COMvError/3(COMv_ref) -> [COMv_ref]
  COMvError/1(PushDetected) -> [PushDetected]

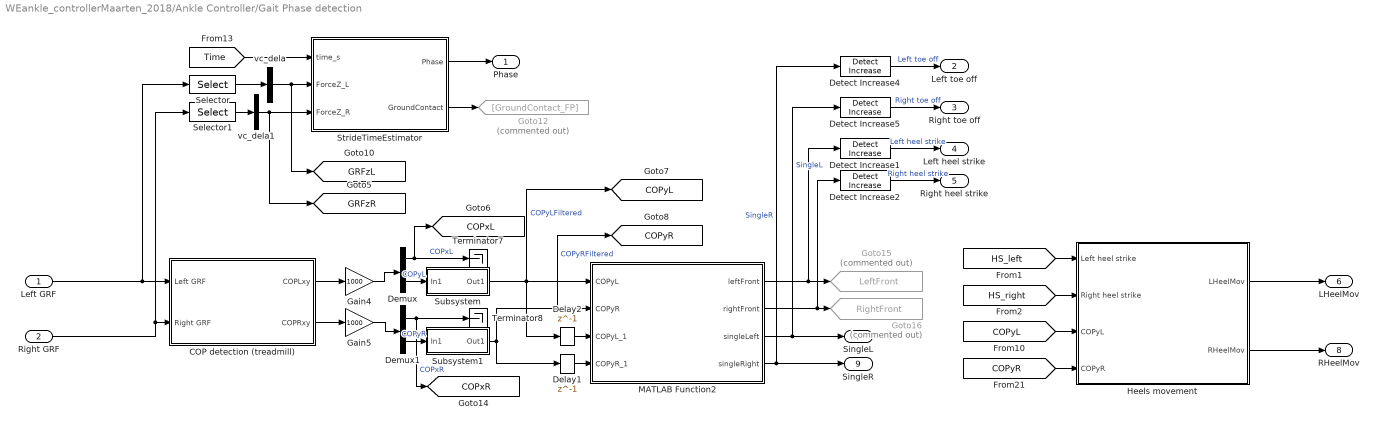
== system WEankle_controllerMaarten_2018/Ankle Controller/Gait Phase detection ==
  Left GRF : Inport
  Right GRF : Inport  Port=2
  COP detection (treadmill) : Subsystem
  Delay1 : Delay  DelayLength=1
  Delay2 : Delay  DelayLength=1
  Demux : Demux  Outputs=2
  Demux1 : Demux  Outputs=2
  Detect Increase{1..2,4..5} (4 alike) : simulink/Logic and Bit Operations/Detect Increase  vinit=0  OutDataTypeStr=boolean
  Gain4 : Gain  Gain=1000
  Gain5 : Gain  Gain=1000
  Goto12 : Goto  Commented=on  GotoTag=GroundContact_FP
  Goto15 : Goto  Commented=on  GotoTag=LeftFront  TagVisibility=global
  Goto16 : Goto  Commented=on  GotoTag=RightFront  TagVisibility=global
  Heels movement : Subsystem
  MATLAB Function2 : MATLAB Function  TreatAsAtomicUnit=on
  Selector : Selector  InputPortWidth=6  IndexOptions=Index vector (dialog)  Indices=3  OutputSizes=1
  Selector1 : Selector  InputPortWidth=6  IndexOptions=Index vector (dialog)  Indices=3  OutputSizes=1
  StrideTimeEstimator : Subsystem
  Subsystem : Subsystem
  Subsystem1 : Subsystem
  Terminator7 : Terminator
  Terminator8 : Terminator
  vc_dela : Concatenate  NumInputs=1
  vc_dela1 : Concatenate  NumInputs=1
  Phase : Outport
  Left toe off : Outport  Port=2
  Right toe off : Outport  Port=3
  Left heel strike : Outport  Port=4
  Right heel strike : Outport  Port=5
  LHeelMov : Outport  Port=6
  SingleL : Outport  Port=7
  RHeelMov : Outport  Port=8
  SingleR : Outport  Port=9
  tag scope: COPxL=global, COPxR=global, COPyL=global, COPyR=global, GRFzL=global, GRFzR=global
  wires:
  Selector1/1 -> vc_dela1/1
  Subsystem/1(Out1) -> [COPyL], Delay2/1, MATLAB Function2/1(COPyL)  "COPyLFiltered"
  [Time] -> StrideTimeEstimator/1(time_s)
  Heels movement/1(LHeelMov) -> LHeelMov/1
  MATLAB Function2/2(rightFront) -> Detect Increase2/1, Goto16/1
  [COPyL] -> Heels movement/3(COPyL)
  vc_dela/1 -> [GRFzL], StrideTimeEstimator/2(ForceZ_L)
  MATLAB Function2/1(leftFront) -> Goto15/1, Detect Increase1/1
  vc_dela1/1 -> [GRFzR], StrideTimeEstimator/3(ForceZ_R)
  Selector/1 -> vc_dela/1
  Detect Increase2/1 -> Right heel strike/1  "Right heel strike"
  Subsystem1/1(Out1) -> [COPyR], MATLAB Function2/2(COPyR), Delay1/1  "COPyRFiltered"
  COP detection (treadmill)/2(COPRxy) -> Gain5/1
  Right GRF/1 -> Selector1/1, COP detection (treadmill)/2(Right GRF)
  Demux/1 -> Terminator7/1, [COPxL]  "COPxL"
  Delay2/1 -> MATLAB Function2/3(COPyL_1)
  Left GRF/1 -> Selector/1, COP detection (treadmill)/1(Left GRF)
  COP detection (treadmill)/1(COPLxy) -> Gain4/1
  Demux1/2 -> Subsystem1/1(In1)  "COPyR"
  Heels movement/2(RHeelMov) -> RHeelMov/1
  Gain5/1 -> Demux1/1
  Detect Increase5/1 -> Right toe off/1  "Right toe off"
  Demux1/1 -> Terminator8/1, [COPxR]  "COPxR"
  [HS_left] -> Heels movement/1(Left heel strike)
  [HS_right] -> Heels movement/2(Right heel strike)
  Gain4/1 -> Demux/1
  StrideTimeEstimator/1(Phase) -> Phase/1
  Delay1/1 -> MATLAB Function2/4(COPyR_1)
  [COPyR] -> Heels movement/4(COPyR)
  Demux/2 -> Subsystem/1(In1)  "COPyL"
  MATLAB Function2/4(singleRight) -> SingleR/1, Detect Increase4/1  "SingleR"
  StrideTimeEstimator/2(GroundContact) -> Goto12/1
  MATLAB Function2/3(singleLeft) -> SingleL/1, Detect Increase5/1  "SingleL"
  Detect Increase4/1 -> Left toe off/1  "Left toe off"
  Detect Increase1/1 -> Left heel strike/1  "Left heel strike"

== system WEankle_controllerMaarten_2018/ForcePlate/Calibration ==
  ForcePlateLeft : Inport
  Start : Inport  Port=2
  ForcePlateRight : Inport  Port=3
  Constant : Constant
  Detect Increase : simulink/Logic and Bit Operations/Detect Increase  vinit=0.0  OutDataTypeStr=boolean
  MATLAB Function : MATLAB Function  TreatAsAtomicUnit=on
  ForcePlateLeft_calib : Outport  VectorParamsAs1DForOutWhenUnconnected=off
  ForcePlateRight_calib : Outport  Port=2  VectorParamsAs1DForOutWhenUnconnected=off
  wires:
  Start/1 -> Detect Increase/1
  ForcePlateLeft/1 -> MATLAB Function/1(left)
  ForcePlateRight/1 -> MATLAB Function/2(right)
  Detect Increase/1 -> MATLAB Function/3(start)
  MATLAB Function/1(left_calib) -> ForcePlateLeft_calib/1
  MATLAB Function/2(right_calib) -> ForcePlateRight_calib/1
  Constant/1 -> MATLAB Function/4(caltime_s)
